simulink model "BuckConverterModel_DCM"  (R2026a)
settings: Solver=ode45  StopTime=0.02

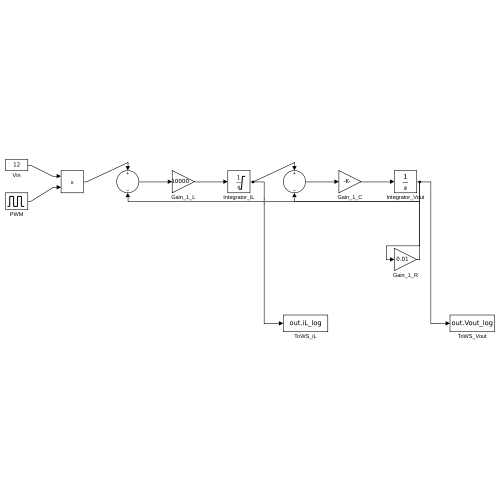
[thumbnail: Simulink's stored preview of the top-level diagram]
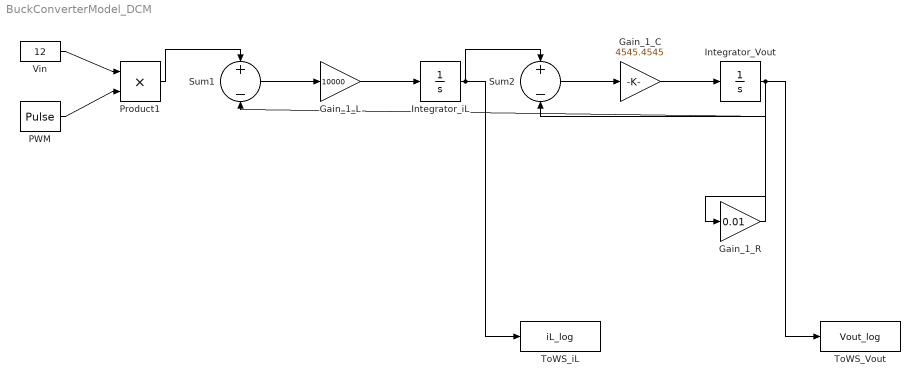
== system BuckConverterModel_DCM ==
  Gain_1_C : Gain  Gain=4545.4545
  Gain_1_L : Gain  Gain=10000
  Gain_1_R : Gain  Gain=0.01
  Integrator_Vout : Integrator
  Integrator_iL : Integrator  LimitOutput=on  LowerSaturationLimit=0
  PWM : DiscretePulseGenerator  PulseType=Time based  Period=1e-05  PulseWidth=41.6667
  Product1 : Product
  Sum1 : Sum  Inputs=+-
  Sum2 : Sum  Inputs=+-
  ToWS_Vout : ToWorkspace  VariableName=Vout_log  SaveFormat=Structure With Time  SampleTime=-1
  ToWS_iL : ToWorkspace  VariableName=iL_log  SaveFormat=Structure With Time  SampleTime=-1
  Vin : Constant  Value=12
  wires:
  Vin/1 -> Product1/1
  PWM/1 -> Product1/2
  Product1/1 -> Sum1/1
  Sum1/1 -> Gain_1_L/1
  Gain_1_L/1 -> Integrator_iL/1
  Integrator_iL/1 -> Sum2/1, ToWS_iL/1
  Sum2/1 -> Gain_1_C/1
  Gain_1_C/1 -> Integrator_Vout/1
  Integrator_Vout/1 -> Sum1/2, Gain_1_R/1, ToWS_Vout/1
  Gain_1_R/1 -> Sum2/2
